simulink library "Surface_Mu_Axle2_LUT_Pos"  (R2024b)
settings: Solver=VariableStepAuto  StartTime=0.0  StopTime=10.0  RelTol=1e-3
undefined symbols (not defined in the file or in its folder): Scene
libraries: Tire_Utilities x4
Description:
  | Simscape Vehicle Templates Library
  | 
  | Copyright 2018-2024 The MathWorks, Inc.
settings Model: Creator=smiller  LastModifiedBy=smiller
settings ModelReferenceCC: EnableRefExpFcnMdlSchedulingChecks=on
settings RTWCC: GPUComputeCapability=3.5

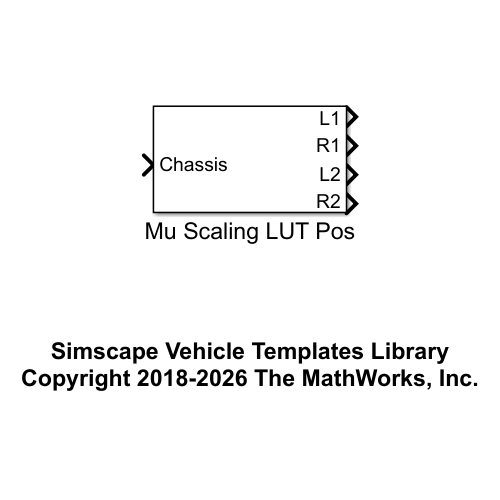
[thumbnail: Simulink's stored preview of the top-level diagram]
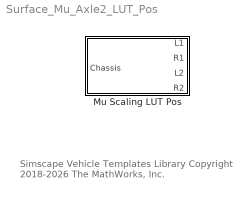
== system Surface_Mu_Axle2_LUT_Pos ==
  note: Simscape Vehicle Templates Library
      | Copyright 2018-2026 The MathWorks, Inc.
  Mu Scaling LUT Pos : Subsystem  VariantControl=Choice  mask(Friction Scaling Coefficient by Position){xposL1=Scene.Mu_Scaling.x, yposL1=Scene.Mu_Scaling.y, ScaleTableL1=Scene.Mu_Scaling.scale, xposR1=Scene.Mu_Scaling.x, yposR1=Scene.Mu_Scaling.y, ScaleTableR1=Scene.Mu_Scaling.scale, xposL2=Scene.Mu_Scaling.x, yposL2=Scene.Mu_Scaling.y, ScaleTableL2=Scene.Mu_Scaling.scale, xposR2=Scene.Mu_Scaling.x, yposR2=Scene.Mu_Scaling.y, ScaleTableR2=Scene.Mu_Scaling.scale}
      mask help: Determines scaling factor for friction coefficient based on wheel x-y position.
      mask TypeOptions xposL1: LUT Scale L1/BreakpointsForDimension1
      mask TypeOptions yposL1: LUT Scale L1/BreakpointsForDimension2
      mask TypeOptions ScaleTableL1: LUT Scale L1/Table
      mask TypeOptions xposR1: LUT Scale R1/BreakpointsForDimension1
      mask TypeOptions yposR1: LUT Scale R1/BreakpointsForDimension2
      mask TypeOptions ScaleTableR1: LUT Scale R1/Table
      mask TypeOptions xposL2: LUT Scale L2/BreakpointsForDimension1
      mask TypeOptions yposL2: LUT Scale L2/BreakpointsForDimension2
      mask TypeOptions ScaleTableL2: LUT Scale L2/Table
      mask TypeOptions xposR2: LUT Scale R2/BreakpointsForDimension1
      mask TypeOptions yposR2: LUT Scale R2/BreakpointsForDimension2
      mask TypeOptions ScaleTableR2: LUT Scale R2/Table
      mask DialogControl text_whl Prompt: Wheel
      mask DialogControl text_xpos Prompt: X [1xm] (m)
      mask DialogControl text_ypos Prompt: Y [1xn] (m)
      mask DialogControl text_mu Prompt: Scale [mxn] (m)
      mask DialogControl text_L1 Prompt: L1
      mask DialogControl text_R1 Prompt: R1
      mask DialogControl text_L2 Prompt: L2
      mask DialogControl text_R2 Prompt: R2

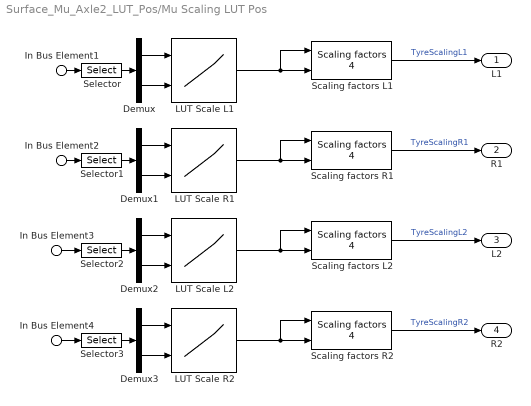
== system Surface_Mu_Axle2_LUT_Pos/Mu Scaling LUT Pos ==
  In Bus Element1 : Inport  PortName=Chassis  Element=WhlL1.xyz
  In Bus Element2 : Inport  PortName=Chassis  Element=WhlR1.xyz
  In Bus Element3 : Inport  PortName=Chassis  Element=WhlL2.xyz
  In Bus Element4 : Inport  PortName=Chassis  Element=WhlR2.xyz
  Demux{,1..3} (4 alike) : Demux  Outputs=2
  LUT Scale L1 : Lookup_n-D  BreakpointsForDimension1=xposL1  BreakpointsForDimension2=yposL1  Table=ScaleTableL1  InternalRulePriority=Speed  RndMeth=Simplest
      settings: InputPortMap=u0,u1
  LUT Scale L2 : Lookup_n-D  BreakpointsForDimension1=xposL2  BreakpointsForDimension2=yposL2  Table=ScaleTableL2  InternalRulePriority=Speed  RndMeth=Simplest
      settings: InputPortMap=u0,u1
  LUT Scale R1 : Lookup_n-D  BreakpointsForDimension1=xposR1  BreakpointsForDimension2=yposR1  Table=ScaleTableR1  InternalRulePriority=Speed  RndMeth=Simplest
      settings: InputPortMap=u0,u1
  LUT Scale R2 : Lookup_n-D  BreakpointsForDimension1=xposR2  BreakpointsForDimension2=yposR2  Table=ScaleTableR2  InternalRulePriority=Speed  RndMeth=Simplest
      settings: InputPortMap=u0,u1
  Scaling factors L1 : Tire_Utilities/Scaling factors 4  LKX=1  LKY=1  LKYC=1  LTR=1  LKZC=1
  Scaling factors L2 : Tire_Utilities/Scaling factors 4  LKX=1  LKY=1  LKYC=1  LTR=1  LKZC=1
  Scaling factors R1 : Tire_Utilities/Scaling factors 4  LKX=1  LKY=1  LKYC=1  LTR=1  LKZC=1
  Scaling factors R2 : Tire_Utilities/Scaling factors 4  LKX=1  LKY=1  LKYC=1  LTR=1  LKZC=1
  Selector{,1..3} (4 alike) : Selector  InputPortWidth=3  IndexOptions=Index vector (dialog)  Indices=[1 2]  OutputSizes=1
  L1 : Outport  VectorParamsAs1DForOutWhenUnconnected=off
  R1 : Outport  Port=2  VectorParamsAs1DForOutWhenUnconnected=off
  L2 : Outport  Port=3  VectorParamsAs1DForOutWhenUnconnected=off
  R2 : Outport  Port=4  VectorParamsAs1DForOutWhenUnconnected=off
  wires:
  In Bus Element1/1 -> Selector/1
  LUT Scale L1/1 -> Scaling factors L1/1, Scaling factors L1/2
  Scaling factors L1/1 -> L1/1  "TyreScalingL1"
  Scaling factors R1/1 -> R1/1  "TyreScalingR1"
  LUT Scale R1/1 -> Scaling factors R1/1, Scaling factors R1/2
  In Bus Element2/1 -> Selector1/1
  LUT Scale L2/1 -> Scaling factors L2/1, Scaling factors L2/2
  Scaling factors L2/1 -> L2/1  "TyreScalingL2"
  Scaling factors R2/1 -> R2/1  "TyreScalingR2"
  LUT Scale R2/1 -> Scaling factors R2/1, Scaling factors R2/2
  Selector/1 -> Demux/1
  Demux/2 -> LUT Scale L1/2
  Demux1/1 -> LUT Scale R1/1
  Demux1/2 -> LUT Scale R1/2
  Selector1/1 -> Demux1/1
  In Bus Element3/1 -> Selector2/1
  Demux2/1 -> LUT Scale L2/1
  Selector2/1 -> Demux2/1
  Demux2/2 -> LUT Scale L2/2
  In Bus Element4/1 -> Selector3/1
  Selector3/1 -> Demux3/1
  Demux3/1 -> LUT Scale R2/1
  Demux3/2 -> LUT Scale R2/2
  Demux/1 -> LUT Scale L1/1
